simulink model "HeadwayControlExperimenting"  (R2018a)
settings: Solver=FixedStepAuto  StartTime=0.0  StopTime=tsim  RelTol=1e-3  EnableMultiTasking=on
values from neighbouring files (symbols this model uses):
  EndVel = (Time2-Time1)*Slope+StartVel    (= 31.525)    [HeadwayControlSimScript.m]    (also in HeadwayControlSimScriptExperiment.m; HeadwayControlSimScriptSimplified.m)
  h = 2    [HeadwayControlSimScript.m]    (also in HeadwayControlSimScriptExperiment.m; HeadwayControlSimScriptSimplified.m)
  InputNum = 3    [HeadwayControlSimScript.m]    (also in HeadwayControlSimScriptExperiment.m; HeadwayControlSimScriptSimplified.m)
  InputTime = 1    [HeadwayControlSimScript.m]    (also in HeadwayControlSimScriptExperiment.m; HeadwayControlSimScriptSimplified.m)
  lambda = 0.001    [HeadwayControlSimScript.m]    (also in HeadwayControlSimScriptExperiment.m = 0.135; HeadwayControlSimScriptSimplified.m)
  Rinit = StartVel*h*4    (= 56)    [HeadwayControlSimScriptExperiment.m]
  Slope = 0.5*g    (= 4.905)    [HeadwayControlSimScript.m]    (also in HeadwayControlSimScriptExperiment.m; HeadwayControlSimScriptSimplified.m)
  StartVel = 7    [HeadwayControlSimScript.m]    (also in HeadwayControlSimScriptExperiment.m; HeadwayControlSimScriptSimplified.m)
  tau = .5    (= 0.5)    [HeadwayControlSimScript.m]    (also in HeadwayControlSimScriptExperiment.m; HeadwayControlSimScriptSimplified.m)
  Vinit = StartVel*1.5    (= 10.5)    [HeadwayControlSimScriptExperiment.m]
libraries: simulink x3
settings Model: SimulationMode=external  Creator=domin  LastModifiedBy=domin
settings SolverCC: PositivePriorityOrder=on
settings OptimizationCC: EnhancedBackFolding=on  PassReuseOutputArgsAs=Individual arguments  MaxStackSize=64  OptimizeBlockOrder=speed  DifferentSizesBufferReuse=on  OptimizationCustomize=off
settings DebuggingCC: ParameterTunabilityLossMsg=error
settings HardwareCC: ProdBitPerPointer=32  ProdBitPerSizeT=32  ProdBitPerPtrDiffT=32  ProdLargestAtomicInteger=Long  ProdLargestAtomicFloat=Double  ProdWordSize=32  ProdHWDeviceType=ARM Compatible->ARM Cortex  UseEmbeddedCoderFeatures=off
settings SFSimCC: MATLABDynamicMemAlloc=off
settings RTWCC: SystemTargetFile=ert.tlc  HardwareBoard=Raspberry Pi  TLCOptions="-aInlineSetEventsForThisBaseRateFcn=TLC_FALSE -aSuppressMultiTaskScheduler=TLC_FALSE  -aRateBasedStepFcn=0"  TemplateMakefile=ert_default_tmf  GenerateReport=on  Toolchain=GNU GCC Raspberry Pi  BuildConfiguration=Faster Runs  IncludeHyperlinkInReport=on  LaunchReport=on  GenerateTraceInfo=on  GenerateTraceReport=on  GenerateTraceReportSl=on  GenerateTraceReportSf=on  GenerateTraceReportEml=on
settings CodeAppCC: ForceParamTrailComments=on  IgnoreCustomStorageClasses=off  OperatorAnnotations=on  SimulinkDataObjDesc=on  SFDataObjDesc=on  InsertBlockDesc=on
settings ERTTargetCC: SupportNonInlinedSFcns=on  SupportVariableSizeSignals=on

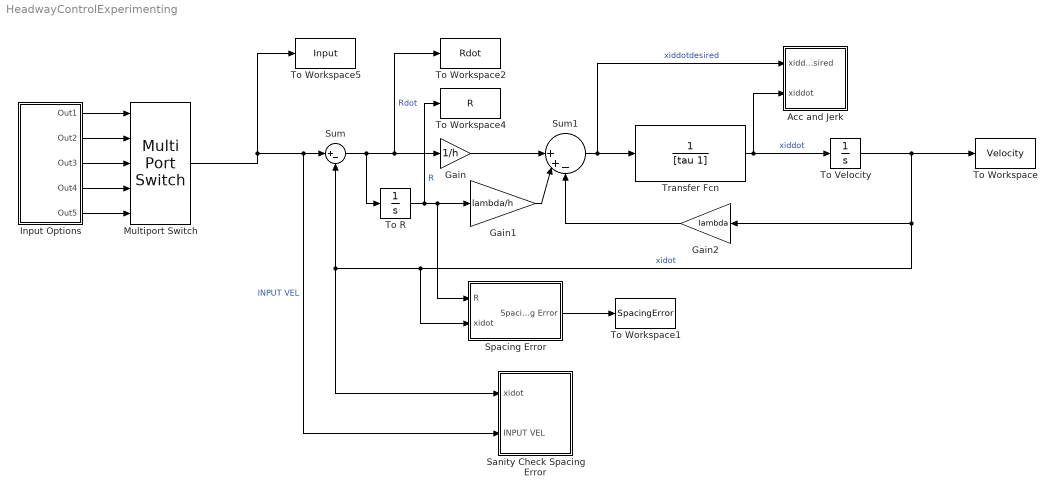
== system HeadwayControlExperimenting ==
  Acc and Jerk : Subsystem
  Gain : Gain  Gain=1/h
  Gain1 : Gain  Gain=lambda/h
  Gain2 : Gain  Gain=lambda
  Input Options : Subsystem
  Multiport Switch : MultiPortSwitch  Inputs=4
  Sanity Check Spacing Error : Subsystem
  Spacing Error : Subsystem
  Sum : Sum  Inputs=|+-
  Sum1 : Sum  Inputs=||++-
  To R : Integrator  InitialCondition=Rinit
  To Velocity : Integrator  InitialCondition=Vinit
  To Workspace : ToWorkspace  VariableName=Velocity  SampleTime=-1
  To Workspace1 : ToWorkspace  VariableName=SpacingError  SampleTime=-1
  To Workspace2 : ToWorkspace  VariableName=Rdot  SampleTime=-1
  To Workspace4 : ToWorkspace  VariableName=R  SampleTime=-1
  To Workspace5 : ToWorkspace  VariableName=Input  SampleTime=-1
  Transfer Fcn : TransferFcn  Denominator=[tau 1]
  wires:
  Gain2/1 -> Sum1/3
  Input Options/4(Out4) -> Multiport Switch/4
  Input Options/3(Out3) -> Multiport Switch/3
  Input Options/1(Out1) -> Multiport Switch/1
  Sum1/1 -> Acc and Jerk/1(xiddotdesired), Transfer Fcn/1  "xiddotdesired"
  Gain/1 -> Sum1/1
  To Velocity/1 -> Spacing Error/2(xidot), Sum/2, Sanity Check Spacing Error/1(xidot), Gain2/1, To Workspace/1  "xidot"
  Spacing Error/1(Spacing Error) -> To Workspace1/1
  Gain1/1 -> Sum1/2
  Multiport Switch/1 -> To Workspace5/1, Sum/1, Sanity Check Spacing Error/2(INPUT VEL)  "INPUT VEL"
  Sum/1 -> To R/1, To Workspace2/1, Gain/1  "Rdot"
  Input Options/2(Out2) -> Multiport Switch/2
  Input Options/5(Out5) -> Multiport Switch/5
  Transfer Fcn/1 -> Acc and Jerk/2(xiddot), To Velocity/1  "xiddot"
  To R/1 -> To Workspace4/1, Spacing Error/1(R), Gain1/1  "R"

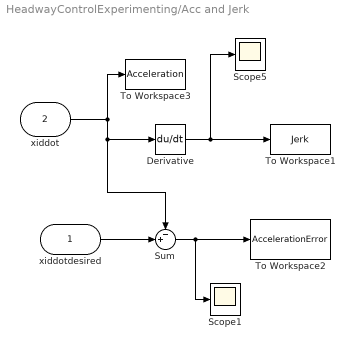
== system HeadwayControlExperimenting/Acc and Jerk ==
  xiddotdesired : Inport
  xiddot : Inport  Port=2
  Derivative : Derivative
  Scope1 : Scope
  Scope5 : Scope
  Sum : Sum  Inputs=-+|
  To Workspace1 : ToWorkspace  VariableName=Jerk  SampleTime=-1
  To Workspace2 : ToWorkspace  VariableName=AccelerationError  SampleTime=-1
  To Workspace3 : ToWorkspace  VariableName=Acceleration  SampleTime=-1
  wires:
  xiddot/1 -> To Workspace3/1, Derivative/1, Sum/1
  Derivative/1 -> To Workspace1/1, Scope5/1
  xiddotdesired/1 -> Sum/2
  Sum/1 -> Scope1/1, To Workspace2/1

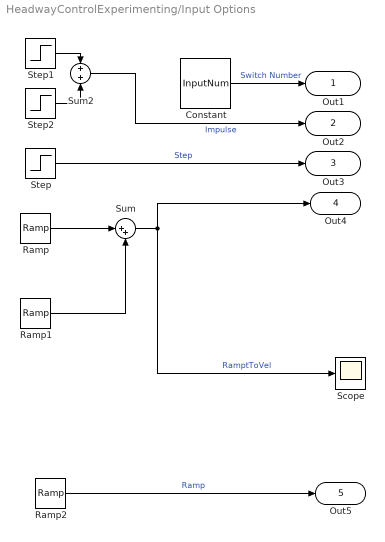
== system HeadwayControlExperimenting/Input Options ==
  Constant : Constant  Value=InputNum
  Ramp : simulink/Sources/Ramp  slope=Slope  start=Time1  InitialOutput=StartVel
  Ramp1 : simulink/Sources/Ramp  slope=-Slope  start=Time2  InitialOutput=0
  Ramp2 : simulink/Sources/Ramp  slope=Slope  start=Time1  InitialOutput=StartVel
  Scope : Scope
  Step : Step  Time=InputTime  Before=StartVel  After=EndVel  SampleTime=0
  Step1 : Step  Time=InputTime  Before=StartVel  After=StartVel+(1*10^10)  SampleTime=0
  Step2 : Step  Time=InputTime + (1*10^-10)  After=-(1*10^10)  SampleTime=0
  Sum : Sum  Inputs=|++
  Sum2 : Sum
  Out1 : Outport
  Out2 : Outport  Port=2
  Out3 : Outport  Port=3
  Out4 : Outport  Port=4
  Out5 : Outport  Port=5
  wires:
  Sum2/1 -> Out2/1  "Impulse"
  Constant/1 -> Out1/1  "Switch Number"
  Step2/1 -> Sum2/2
  Step1/1 -> Sum2/1
  Step/1 -> Out3/1  "Step"
  Ramp/1 -> Sum/1
  Ramp1/1 -> Sum/2
  Sum/1 -> Out4/1, Scope/1  "RamptToVel"
  Ramp2/1 -> Out5/1  "Ramp"

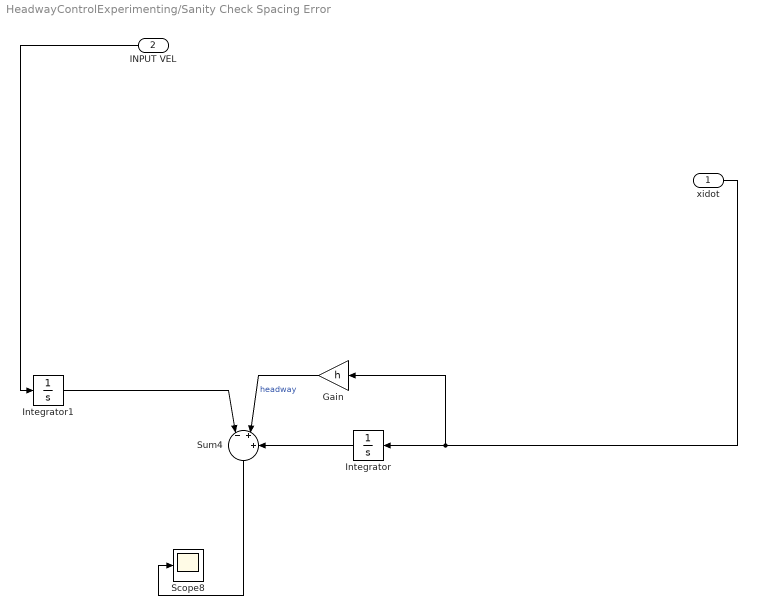
== system HeadwayControlExperimenting/Sanity Check Spacing Error ==
  xidot : Inport
  INPUT VEL : Inport  Port=2
  Gain : Gain  Gain=h
  Integrator : Integrator
  Integrator1 : Integrator  InitialCondition=h*StartVel
  Scope8 : Scope
  Sum4 : Sum  Inputs=|-++
  wires:
  Integrator/1 -> Sum4/3
  Integrator1/1 -> Sum4/1
  xidot/1 -> Gain/1, Integrator/1
  INPUT VEL/1 -> Integrator1/1
  Sum4/1 -> Scope8/1
  Gain/1 -> Sum4/2  "headway"

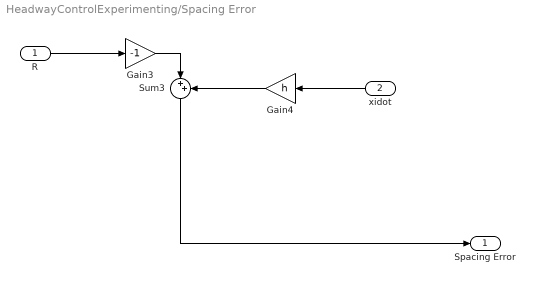
== system HeadwayControlExperimenting/Spacing Error ==
  R : Inport
  xidot : Inport  Port=2
  Gain3 : Gain  Gain=-1
  Gain4 : Gain  Gain=h
  Sum3 : Sum  Inputs=|++
  Spacing Error : Outport
  wires:
  Sum3/1 -> Spacing Error/1
  R/1 -> Gain3/1
  xidot/1 -> Gain4/1
  Gain3/1 -> Sum3/1
  Gain4/1 -> Sum3/2
